simulink model "Copy_of_CT_mod1"  (Simulink 7.9)
settings: Solver=ode15s  StartTime=0.0  StopTime=simu.trantime  RelTol=1e-7
values from neighbouring files (symbols this model uses):
  OSR = 64    [MakeModulator_CT.m]
undefined symbols (not defined in the file or in its folder): dc, Fs, mod, sinamp, sinfreq
libraries: dsparch4 x1, simulink x1, dspsrcs4 x1
settings Model: Creator=Isacco Arnaldi  LastModifiedBy=Arnaldi Isacco
settings SolverCC: MaxOrder=3  SolverResetMethod=Robust  AutoInsertRateTranBlk=on
settings DataIOCC: MaxDataPoints=50000  SaveOutput=off  SaveTime=off
settings DebuggingCC: StrictBusMsg=Warning
settings CodeAppCC: CustomSymbolStrType=$N$R$M_T
settings GRTTargetCC: CombineOutputUpdateFcns=off  GRTInterface=on

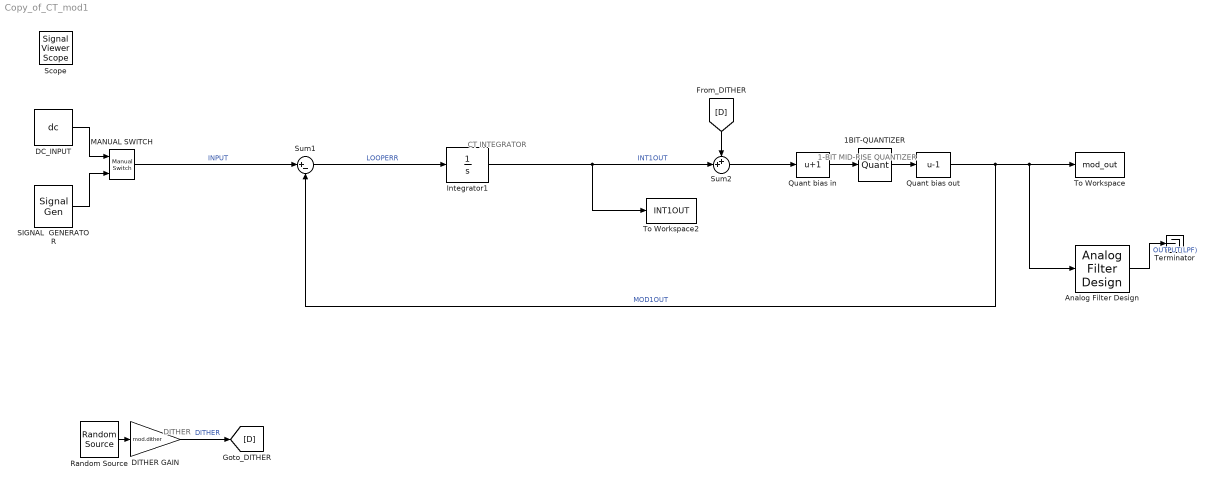
== system Copy_of_CT_mod1 ==
  note: 1-BIT MID-RISE QUANTIZER
  note: DITHER
  note: CT INTEGRATOR
  1BIT-QUANTIZER : Quantizer  QuantizationInterval=2  LinearizeAsGain=off  SampleTime=1/Fs
      settings: AttributesFormatString=step = 2
  Analog Filter Design : dsparch4/Analog Filter Design  method=Butterworth  filttype=Lowpass  N=8  Wlo=pi*(Fs/OSR)  Whi=80  Rp=2  Rs=40
      settings: AttributesFormatString=Low-pass filter the loop output\nto illustrate intuitively how the\npulse density modulated +1/-1\noutput stream does indeed capture\nthe input signal
  DC_INPUT : Constant  Value=dc  VectorParams1D=off  OutDataTypeStr=double  SampleTime=1/Fs
  DITHER GAIN : Gain  Gain=mod.dither  SampleTime=1/Fs
  Integrator1 : Integrator  LimitOutput=on  IgnoreLimit=on
  MANUAL SWITCH : simulink/Signal Routing/Manual Switch  sw=0  action=0  varsize=off
      settings: AttributesFormatString=Double click to\nselect the desired\ninput
  Quant bias in : Bias  Bias=1
      settings: AttributesFormatString=Need offset to give\nMID-RISE quantiser
  Quant bias out : Bias  Bias=-1
      settings: AttributesFormatString=Shift outputs to\n..., -2, 1, 1, ...
  Random Source : dspsrcs4/Random Source  SrcType=Uniform  NormMethod=Ziggurat  CltLength=12  MinVal=-1  MaxVal=1  MeanVal=0  VarVal=1  RepMode=Not repeatable  rawSeed=1  IsInherit=off  SampMode=Discrete  SampTime=1/Fs  SampFrame=1  DataType=Double  OutComplex=Real
  SIGNAL  GENERATOR : SignalGenerator  Amplitude=sinamp  Frequency=sinfreq  VectorParams1D=off
  Sum1 : Sum  Inputs=|+-  SampleTime=1/Fs
      settings: AttributesFormatString=Modulator Input\nLoop Error (input - fbk)
  Sum2 : Sum  Inputs=++|
  Terminator : Terminator
  To Workspace : ToWorkspace  VariableName=mod_out  SampleTime=-1
      settings: AttributesFormatString=Export output to\nworkspace for\npost-processing
  To Workspace2 : ToWorkspace  VariableName=INT1OUT  SampleTime=-1
      settings: AttributesFormatString=Export output to\nworkspace for\npost-processing
  Scope : SignalViewerScope  IOType=viewer  NumInputPorts=4  ZoomMode=xonly  RefreshTime=0.019600
      settings: YMin=-0.75~-2~-7.5e-07~0  YMax=0.75~2~7.5e-07~1
  wires:
  Random Source/1 -> DITHER GAIN/1
  Quant bias out/1 -> To Workspace/1, Analog Filter Design/1, Sum1/2  "MOD1OUT"
  DITHER GAIN/1 -> [D]  "DITHER"
  DC_INPUT/1 -> MANUAL SWITCH/1
  SIGNAL  GENERATOR/1 -> MANUAL SWITCH/2
  MANUAL SWITCH/1 -> Sum1/1  "INPUT"
  Analog Filter Design/1 -> Terminator/1  "OUTPUT(LPF)"
  Sum2/1 -> Quant bias in/1
  [D] -> Sum2/1
  Integrator1/1 -> To Workspace2/1, Sum2/2  "INT1OUT"
  Sum1/1 -> Integrator1/1  "LOOPERR"
  1BIT-QUANTIZER/1 -> Quant bias out/1
  Quant bias in/1 -> 1BIT-QUANTIZER/1
